simulink library "Displays_Lib"  (Simulink 8.1)
settings: Solver=ode45  StartTime=0.0  StopTime=10.0  RelTol=1e-3
undefined symbols (not defined in the file): ending_column_index, ending_row_index, framebuffer_16x1, framebuffer_2x2, framebuffer_4x4, framebuffer_8x8, HEIGHT, hot, POS_X, POS_Y, starting_column_index, starting_row_index, WIDTH
libraries: dspmtrx3 x119, commutil2 x100, dspsnks4 x4
(part 1 of 2)
settings Model: Creator=uzivatel  LastModifiedBy=uzivatel

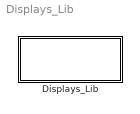
== system Displays_Lib ==
  Displays_Lib : Subsystem

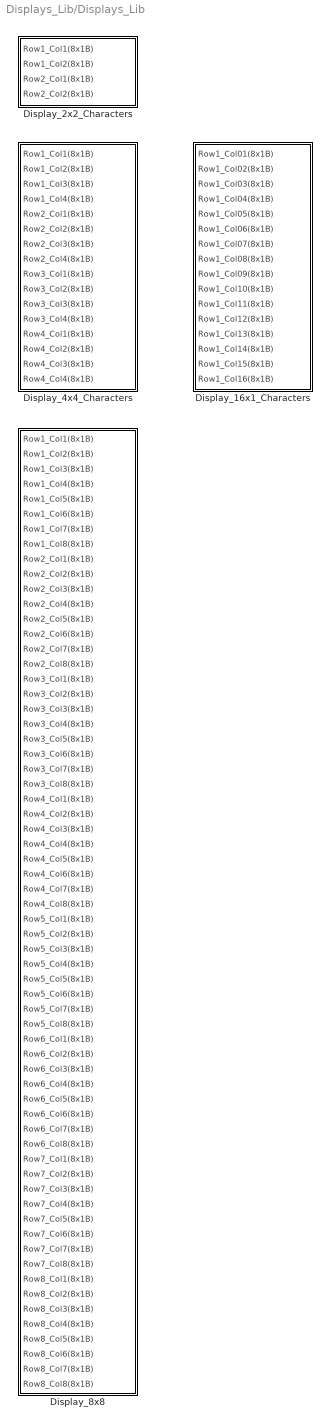
== system Displays_Lib/Displays_Lib ==
  Display_16x1_Characters : Subsystem
  Display_2x2_Characters : Subsystem
  Display_4x4_Characters : Subsystem
  Display_8x8 : Subsystem

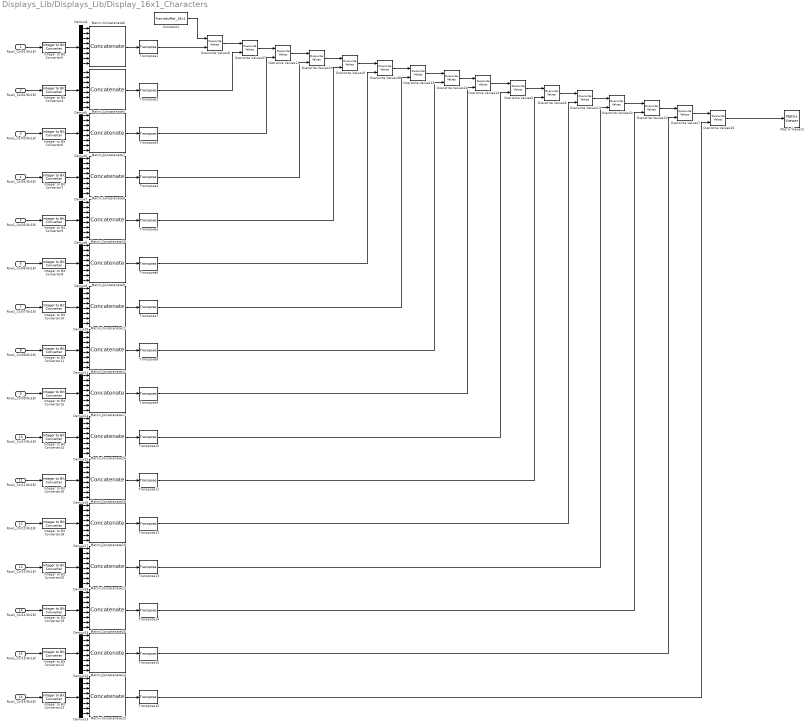
== system Displays_Lib/Displays_Lib/Display_16x1_Characters ==
  Row1_Col01(8x1B) : Inport
  Row1_Col02(8x1B) : Inport  Port=2
  Row1_Col03(8x1B) : Inport  Port=3
  Row1_Col04(8x1B) : Inport  Port=4
  Row1_Col05(8x1B) : Inport  Port=5
  Row1_Col06(8x1B) : Inport  Port=6
  Row1_Col07(8x1B) : Inport  Port=7
  Row1_Col08(8x1B) : Inport  Port=8
  Row1_Col09(8x1B) : Inport  Port=9
  Row1_Col10(8x1B) : Inport  Port=10
  Row1_Col11(8x1B) : Inport  Port=11
  Row1_Col12(8x1B) : Inport  Port=12
  Row1_Col13(8x1B) : Inport  Port=13
  Row1_Col14(8x1B) : Inport  Port=14
  Row1_Col15(8x1B) : Inport  Port=15
  Row1_Col16(8x1B) : Inport  Port=16
  Constant1 : Constant  Value=framebuffer_16x1  OutDataTypeStr=uint8
  Demux{4..19} (16 alike) : Demux  Outputs=8
  Integer to Bit Converter{4..16,18..20} (16 alike) : commutil2/Integer to Bit Converter  nbits=8  signedInputValues=Unsigned  bitOrder=MSB first  outDtype=uint8
  Matrix Concatenate{5..20} (16 alike) : Concatenate  NumInputs=8  Mode=Multidimensional array  ConcatenateDimension=2
  Matrix Viewer2 : dspsnks4/Matrix Viewer  ImageParams=off  CMapStr=[0 0.3 0; 0 1 0]  AxisColorbar=on  AxisParams=off  AxisOrigin=Upper left corner  XLabel=X-axis  YLabel=Y-axis  ZLabel=Z-axis  FigPos=[POS_X POS_Y-140 WIDTH HEIGHT]  AxisZoom=on
      settings: YMin=0  YMax=1
  Overwrite Values10 : dspmtrx3/Overwrite Values  OverWriteDiag=Submatrix  valFrom2ndIP=Second input port  ConstValue=0  RowSpan=Range of rows  RowStartMode=Index  RowStartIndex=starting_row_index(1)  RowEndMode=Index  RowEndIndex=ending_row_index(1)  ColSpan=Range of columns  ColStartMode=Index  ColStartIndex=starting_column_index(14)  ColEndMode=Index  ColEndIndex=ending_column_index(14)  DiagSpan=Range of elements  DiagStartMode=Index  DiagStartIndex=2  DiagEndMode=Index  DiagEndIndex=4
  Overwrite Values11 : dspmtrx3/Overwrite Values  OverWriteDiag=Submatrix  valFrom2ndIP=Second input port  ConstValue=0  RowSpan=Range of rows  RowStartMode=Index  RowStartIndex=starting_row_index(1)  RowEndMode=Index  RowEndIndex=ending_row_index(1)  ColSpan=Range of columns  ColStartMode=Index  ColStartIndex=starting_column_index(3)  ColEndMode=Index  ColEndIndex=ending_column_index(3)  DiagSpan=Range of elements  DiagStartMode=Index  DiagStartIndex=2  DiagEndMode=Index  DiagEndIndex=4
  Overwrite Values12 : dspmtrx3/Overwrite Values  OverWriteDiag=Submatrix  valFrom2ndIP=Second input port  ConstValue=0  RowSpan=Range of rows  RowStartMode=Index  RowStartIndex=starting_row_index(1)  RowEndMode=Index  RowEndIndex=ending_row_index(1)  ColSpan=Range of columns  ColStartMode=Index  ColStartIndex=starting_column_index(7)  ColEndMode=Index  ColEndIndex=ending_column_index(7)  DiagSpan=Range of elements  DiagStartMode=Index  DiagStartIndex=2  DiagEndMode=Index  DiagEndIndex=4
  Overwrite Values13 : dspmtrx3/Overwrite Values  OverWriteDiag=Submatrix  valFrom2ndIP=Second input port  ConstValue=0  RowSpan=Range of rows  RowStartMode=Index  RowStartIndex=starting_row_index(1)  RowEndMode=Index  RowEndIndex=ending_row_index(1)  ColSpan=Range of columns  ColStartMode=Index  ColStartIndex=starting_column_index(12)  ColEndMode=Index  ColEndIndex=ending_column_index(12)  DiagSpan=Range of elements  DiagStartMode=Index  DiagStartIndex=2  DiagEndMode=Index  DiagEndIndex=4
  Overwrite Values14 : dspmtrx3/Overwrite Values  OverWriteDiag=Submatrix  valFrom2ndIP=Second input port  ConstValue=0  RowSpan=Range of rows  RowStartMode=Index  RowStartIndex=starting_row_index(1)  RowEndMode=Index  RowEndIndex=ending_row_index(1)  ColSpan=Range of columns  ColStartMode=Index  ColStartIndex=starting_column_index(9)  ColEndMode=Index  ColEndIndex=ending_column_index(9)  DiagSpan=Range of elements  DiagStartMode=Index  DiagStartIndex=2  DiagEndMode=Index  DiagEndIndex=4
  Overwrite Values16 : dspmtrx3/Overwrite Values  OverWriteDiag=Submatrix  valFrom2ndIP=Second input port  ConstValue=0  RowSpan=Range of rows  RowStartMode=Index  RowStartIndex=starting_row_index(1)  RowEndMode=Index  RowEndIndex=ending_row_index(1)  ColSpan=Range of columns  ColStartMode=Index  ColStartIndex=starting_column_index(16)  ColEndMode=Index  ColEndIndex=ending_column_index(16)  DiagSpan=Range of elements  DiagStartMode=Index  DiagStartIndex=2  DiagEndMode=Index  DiagEndIndex=4
  Overwrite Values20 : dspmtrx3/Overwrite Values  OverWriteDiag=Submatrix  valFrom2ndIP=Second input port  ConstValue=0  RowSpan=Range of rows  RowStartMode=Index  RowStartIndex=starting_row_index(1)  RowEndMode=Index  RowEndIndex=ending_row_index(1)  ColSpan=Range of columns  ColStartMode=Index  ColStartIndex=starting_column_index(13)  ColEndMode=Index  ColEndIndex=ending_column_index(13)  DiagSpan=Range of elements  DiagStartMode=Index  DiagStartIndex=2  DiagEndMode=Index  DiagEndIndex=4
  Overwrite Values23 : dspmtrx3/Overwrite Values  OverWriteDiag=Submatrix  valFrom2ndIP=Second input port  ConstValue=0  RowSpan=Range of rows  RowStartMode=Index  RowStartIndex=starting_row_index(1)  RowEndMode=Index  RowEndIndex=ending_row_index(1)  ColSpan=Range of columns  ColStartMode=Index  ColStartIndex=starting_column_index(4)  ColEndMode=Index  ColEndIndex=ending_column_index(4)  DiagSpan=Range of elements  DiagStartMode=Index  DiagStartIndex=2  DiagEndMode=Index  DiagEndIndex=4
  Overwrite Values24 : dspmtrx3/Overwrite Values  OverWriteDiag=Submatrix  valFrom2ndIP=Second input port  ConstValue=0  RowSpan=Range of rows  RowStartMode=Index  RowStartIndex=starting_row_index(1)  RowEndMode=Index  RowEndIndex=ending_row_index(1)  ColSpan=Range of columns  ColStartMode=Index  ColStartIndex=starting_column_index(8)  ColEndMode=Index  ColEndIndex=ending_column_index(8)  DiagSpan=Range of elements  DiagStartMode=Index  DiagStartIndex=2  DiagEndMode=Index  DiagEndIndex=4
  Overwrite Values37 : dspmtrx3/Overwrite Values  OverWriteDiag=Submatrix  valFrom2ndIP=Second input port  ConstValue=0  RowSpan=Range of rows  RowStartMode=Index  RowStartIndex=starting_row_index(1)  RowEndMode=Index  RowEndIndex=ending_row_index(1)  ColSpan=Range of columns  ColStartMode=Index  ColStartIndex=starting_column_index(2)  ColEndMode=Index  ColEndIndex=ending_column_index(2)  DiagSpan=Range of elements  DiagStartMode=Index  DiagStartIndex=2  DiagEndMode=Index  DiagEndIndex=4
  Overwrite Values38 : dspmtrx3/Overwrite Values  OverWriteDiag=Submatrix  valFrom2ndIP=Second input port  ConstValue=0  RowSpan=Range of rows  RowStartMode=Index  RowStartIndex=starting_row_index(1)  RowEndMode=Index  RowEndIndex=ending_row_index(1)  ColSpan=Range of columns  ColStartMode=Index  ColStartIndex=starting_column_index(6)  ColEndMode=Index  ColEndIndex=ending_column_index(6)  DiagSpan=Range of elements  DiagStartMode=Index  DiagStartIndex=2  DiagEndMode=Index  DiagEndIndex=4
  Overwrite Values5 : dspmtrx3/Overwrite Values  OverWriteDiag=Submatrix  valFrom2ndIP=Second input port  ConstValue=0  RowSpan=Range of rows  RowStartMode=Index  RowStartIndex=starting_row_index(1)  RowEndMode=Index  RowEndIndex=ending_row_index(1)  ColSpan=Range of columns  ColStartMode=Index  ColStartIndex=starting_column_index(10)  ColEndMode=Index  ColEndIndex=ending_column_index(10)  DiagSpan=Range of elements  DiagStartMode=Index  DiagStartIndex=2  DiagEndMode=Index  DiagEndIndex=4
  Overwrite Values6 : dspmtrx3/Overwrite Values  OverWriteDiag=Submatrix  valFrom2ndIP=Second input port  ConstValue=0  RowSpan=Range of rows  RowStartMode=Index  RowStartIndex=starting_row_index(1)  RowEndMode=Index  RowEndIndex=ending_row_index(1)  ColSpan=Range of columns  ColStartMode=Index  ColStartIndex=starting_column_index(11)  ColEndMode=Index  ColEndIndex=ending_column_index(11)  DiagSpan=Range of elements  DiagStartMode=Index  DiagStartIndex=2  DiagEndMode=Index  DiagEndIndex=4
  Overwrite Values7 : dspmtrx3/Overwrite Values  OverWriteDiag=Submatrix  valFrom2ndIP=Second input port  ConstValue=0  RowSpan=Range of rows  RowStartMode=Index  RowStartIndex=starting_row_index(1)  RowEndMode=Index  RowEndIndex=ending_row_index(1)  ColSpan=Range of columns  ColStartMode=Index  ColStartIndex=starting_column_index(15)  ColEndMode=Index  ColEndIndex=ending_column_index(15)  DiagSpan=Range of elements  DiagStartMode=Index  DiagStartIndex=2  DiagEndMode=Index  DiagEndIndex=4
  Overwrite Values8 : dspmtrx3/Overwrite Values  OverWriteDiag=Submatrix  valFrom2ndIP=Second input port  ConstValue=0  RowSpan=Range of rows  RowStartMode=Index  RowStartIndex=starting_row_index(1)  RowEndMode=Index  RowEndIndex=ending_row_index(1)  ColSpan=Range of columns  ColStartMode=Index  ColStartIndex=starting_column_index(1)  ColEndMode=Index  ColEndIndex=ending_column_index(1)  DiagSpan=Range of elements  DiagStartMode=Index  DiagStartIndex=2  DiagEndMode=Index  DiagEndIndex=4
  Overwrite Values9 : dspmtrx3/Overwrite Values  OverWriteDiag=Submatrix  valFrom2ndIP=Second input port  ConstValue=0  RowSpan=Range of rows  RowStartMode=Index  RowStartIndex=starting_row_index(1)  RowEndMode=Index  RowEndIndex=ending_row_index(1)  ColSpan=Range of columns  ColStartMode=Index  ColStartIndex=starting_column_index(5)  ColEndMode=Index  ColEndIndex=ending_column_index(5)  DiagSpan=Range of elements  DiagStartMode=Index  DiagStartIndex=2  DiagEndMode=Index  DiagEndIndex=4
  Transpose{1..16} (16 alike) : dspmtrx3/Transpose  Hermitian=off  overflowFlag=off
  wires:
  Overwrite Values7/1 -> Overwrite Values16/1
  Transpose11/1 -> Overwrite Values6/2
  Transpose13/1 -> Overwrite Values20/2
  Transpose12/1 -> Overwrite Values13/2
  Demux8/8 -> Matrix Concatenate10/8
  Row1_Col05(8x1B)/1 -> Integer to Bit Converter9/1
  Integer to Bit Converter9/1 -> Demux8/1
  Demux9/4 -> Matrix Concatenate9/4
  Integer to Bit Converter11/1 -> Demux11/1
  Demux10/6 -> Matrix Concatenate11/6
  Row1_Col06(8x1B)/1 -> Integer to Bit Converter8/1
  Demux9/7 -> Matrix Concatenate9/7
  Demux11/1 -> Matrix Concatenate12/1
  Demux10/4 -> Matrix Concatenate11/4
  Demux9/2 -> Matrix Concatenate9/2
  Demux11/7 -> Matrix Concatenate12/7
  Demux10/8 -> Matrix Concatenate11/8
  Demux11/4 -> Matrix Concatenate12/4
  Demux9/5 -> Matrix Concatenate9/5
  Demux11/2 -> Matrix Concatenate12/2
  Demux11/5 -> Matrix Concatenate12/5
  Demux11/6 -> Matrix Concatenate12/6
  Row1_Col08(8x1B)/1 -> Integer to Bit Converter11/1
  Demux10/3 -> Matrix Concatenate11/3
  Demux8/2 -> Matrix Concatenate10/2
  Demux8/7 -> Matrix Concatenate10/7
  Overwrite Values24/1 -> Overwrite Values14/1
  Demux10/1 -> Matrix Concatenate11/1
  Demux9/6 -> Matrix Concatenate9/6
  Row1_Col07(8x1B)/1 -> Integer to Bit Converter10/1
  Demux9/8 -> Matrix Concatenate9/8
  Demux10/7 -> Matrix Concatenate11/7
  Demux9/3 -> Matrix Concatenate9/3
  Demux10/2 -> Matrix Concatenate11/2
  Demux11/8 -> Matrix Concatenate12/8
  Demux8/1 -> Matrix Concatenate10/1
  Integer to Bit Converter8/1 -> Demux9/1
  Demux8/5 -> Matrix Concatenate10/5
  Integer to Bit Converter10/1 -> Demux10/1
  Demux11/3 -> Matrix Concatenate12/3
  Demux10/5 -> Matrix Concatenate11/5
  Demux8/6 -> Matrix Concatenate10/6
  Demux8/4 -> Matrix Concatenate10/4
  Demux8/3 -> Matrix Concatenate10/3
  Demux9/1 -> Matrix Concatenate9/1
  Transpose2/1 -> Overwrite Values37/2
  Transpose16/1 -> Overwrite Values16/2
  Transpose14/1 -> Overwrite Values10/2
  Transpose15/1 -> Overwrite Values7/2
  Overwrite Values9/1 -> Overwrite Values38/1
  Overwrite Values6/1 -> Overwrite Values13/1
  Overwrite Values38/1 -> Overwrite Values12/1
  Overwrite Values12/1 -> Overwrite Values24/1
  Overwrite Values14/1 -> Overwrite Values5/1
  Transpose10/1 -> Overwrite Values5/2
  Overwrite Values10/1 -> Overwrite Values7/1
  Integer to Bit Converter18/1 -> Demux17/1
  Transpose5/1 -> Overwrite Values9/2
  Transpose7/1 -> Overwrite Values12/2
  Transpose9/1 -> Overwrite Values14/2
  Transpose4/1 -> Overwrite Values23/2
  Transpose3/1 -> Overwrite Values11/2
  Overwrite Values5/1 -> Overwrite Values6/1
  Overwrite Values20/1 -> Overwrite Values10/1
  Overwrite Values8/1 -> Overwrite Values37/1
  Transpose8/1 -> Overwrite Values24/2
  Demux15/2 -> Matrix Concatenate16/2
  Demux14/3 -> Matrix Concatenate17/3
  Transpose6/1 -> Overwrite Values38/2
  Demux16/1 -> Matrix Concatenate18/1
  Demux15/3 -> Matrix Concatenate16/3
  Overwrite Values11/1 -> Overwrite Values23/1
  Demux15/7 -> Matrix Concatenate16/7
  Demux16/4 -> Matrix Concatenate18/4
  Integer to Bit Converter16/1 -> Demux16/1
  Demux14/1 -> Matrix Concatenate17/1
  Demux15/6 -> Matrix Concatenate16/6
  Demux16/3 -> Matrix Concatenate18/3
  Demux14/4 -> Matrix Concatenate17/4
  Demux16/7 -> Matrix Concatenate18/7
  Demux17/6 -> Matrix Concatenate19/6
  Demux15/5 -> Matrix Concatenate16/5
  Demux14/2 -> Matrix Concatenate17/2
  Demux16/6 -> Matrix Concatenate18/6
  Demux17/7 -> Matrix Concatenate19/7
  Demux16/2 -> Matrix Concatenate18/2
  Demux17/4 -> Matrix Concatenate19/4
  Integer to Bit Converter14/1 -> Demux15/1
  Demux16/5 -> Matrix Concatenate18/5
  Demux15/4 -> Matrix Concatenate16/4
  Demux15/1 -> Matrix Concatenate16/1
  Demux17/5 -> Matrix Concatenate19/5
  Demux19/7 -> Matrix Concatenate20/7
  Integer to Bit Converter19/1 -> Demux19/1
  Demux18/1 -> Matrix Concatenate13/1
  Demux18/2 -> Matrix Concatenate13/2
  Demux18/3 -> Matrix Concatenate13/3
  Demux18/4 -> Matrix Concatenate13/4
  Demux18/5 -> Matrix Concatenate13/5
  Demux18/6 -> Matrix Concatenate13/6
  Demux18/7 -> Matrix Concatenate13/7
  Demux18/8 -> Matrix Concatenate13/8
  Integer to Bit Converter20/1 -> Demux18/1
  Row1_Col13(8x1B)/1 -> Integer to Bit Converter20/1
  Row1_Col15(8x1B)/1 -> Integer to Bit Converter12/1
  Row1_Col14(8x1B)/1 -> Integer to Bit Converter19/1
  Row1_Col16(8x1B)/1 -> Integer to Bit Converter13/1
  Demux17/8 -> Matrix Concatenate19/8
  Demux16/8 -> Matrix Concatenate18/8
  Demux15/8 -> Matrix Concatenate16/8
  Demux17/1 -> Matrix Concatenate19/1
  Demux17/2 -> Matrix Concatenate19/2
  Demux17/3 -> Matrix Concatenate19/3
  Demux19/6 -> Matrix Concatenate20/6
  Demux13/8 -> Matrix Concatenate15/8
  Demux12/8 -> Matrix Concatenate14/8
  Demux19/8 -> Matrix Concatenate20/8
  Demux13/1 -> Matrix Concatenate15/1
  Demux13/2 -> Matrix Concatenate15/2
  Demux13/3 -> Matrix Concatenate15/3
  Demux13/4 -> Matrix Concatenate15/4
  Demux13/5 -> Matrix Concatenate15/5
  Demux13/6 -> Matrix Concatenate15/6
  Demux13/7 -> Matrix Concatenate15/7
  Integer to Bit Converter13/1 -> Demux13/1
  Demux12/1 -> Matrix Concatenate14/1
  Demux12/2 -> Matrix Concatenate14/2
  Demux12/3 -> Matrix Concatenate14/3
  Demux12/4 -> Matrix Concatenate14/4
  Demux12/5 -> Matrix Concatenate14/5
  Demux12/6 -> Matrix Concatenate14/6
  Demux12/7 -> Matrix Concatenate14/7
  Integer to Bit Converter12/1 -> Demux12/1
  Demux19/1 -> Matrix Concatenate20/1
  Demux19/2 -> Matrix Concatenate20/2
  Demux19/3 -> Matrix Concatenate20/3
  Demux19/4 -> Matrix Concatenate20/4
  Demux19/5 -> Matrix Concatenate20/5
  Overwrite Values13/1 -> Overwrite Values20/1
  Demux14/6 -> Matrix Concatenate17/6
  Overwrite Values16/1 -> Matrix Viewer2/1
  Row1_Col09(8x1B)/1 -> Integer to Bit Converter15/1
  Row1_Col11(8x1B)/1 -> Integer to Bit Converter16/1
  Demux14/8 -> Matrix Concatenate17/8
  Constant1/1 -> Overwrite Values8/1
  Row1_Col10(8x1B)/1 -> Integer to Bit Converter14/1
  Demux14/5 -> Matrix Concatenate17/5
  Demux14/7 -> Matrix Concatenate17/7
  Integer to Bit Converter15/1 -> Demux14/1
  Transpose1/1 -> Overwrite Values8/2
  Row1_Col12(8x1B)/1 -> Integer to Bit Converter18/1
  Demux6/2 -> Matrix Concatenate7/2
  Demux6/4 -> Matrix Concatenate7/4
  Demux6/3 -> Matrix Concatenate7/3
  Integer to Bit Converter5/1 -> Demux4/1
  Demux6/1 -> Matrix Concatenate7/1
  Demux6/5 -> Matrix Concatenate7/5
  Demux6/6 -> Matrix Concatenate7/6
  Demux6/7 -> Matrix Concatenate7/7
  Demux4/2 -> Matrix Concatenate6/2
  Row1_Col01(8x1B)/1 -> Integer to Bit Converter5/1
  Integer to Bit Converter7/1 -> Demux7/1
  Demux7/4 -> Matrix Concatenate8/4
  Demux4/4 -> Matrix Concatenate6/4
  Integer to Bit Converter6/1 -> Demux6/1
  Demux4/8 -> Matrix Concatenate6/8
  Demux4/1 -> Matrix Concatenate6/1
  Integer to Bit Converter4/1 -> Demux5/1
  Demux4/7 -> Matrix Concatenate6/7
  Demux4/6 -> Matrix Concatenate6/6
  Demux4/5 -> Matrix Concatenate6/5
  Row1_Col02(8x1B)/1 -> Integer to Bit Converter4/1
  Demux5/4 -> Matrix Concatenate5/4
  Demux5/3 -> Matrix Concatenate5/3
  Demux5/6 -> Matrix Concatenate5/6
  Demux5/8 -> Matrix Concatenate5/8
  Demux5/1 -> Matrix Concatenate5/1
  Demux7/7 -> Matrix Concatenate8/7
  Demux5/2 -> Matrix Concatenate5/2
  Demux7/2 -> Matrix Concatenate8/2
  Demux7/3 -> Matrix Concatenate8/3
  Demux7/8 -> Matrix Concatenate8/8
  Demux6/8 -> Matrix Concatenate7/8
  Demux7/5 -> Matrix Concatenate8/5
  Demux7/6 -> Matrix Concatenate8/6
  Demux7/1 -> Matrix Concatenate8/1
  Demux5/5 -> Matrix Concatenate5/5
  Demux4/3 -> Matrix Concatenate6/3
  Demux5/7 -> Matrix Concatenate5/7
  Row1_Col04(8x1B)/1 -> Integer to Bit Converter7/1
  Row1_Col03(8x1B)/1 -> Integer to Bit Converter6/1
  Overwrite Values23/1 -> Overwrite Values9/1
  Overwrite Values37/1 -> Overwrite Values11/1
  Matrix Concatenate6/1 -> Transpose1/1
  Matrix Concatenate5/1 -> Transpose2/1
  Matrix Concatenate7/1 -> Transpose3/1
  Matrix Concatenate8/1 -> Transpose4/1
  Matrix Concatenate10/1 -> Transpose5/1
  Matrix Concatenate9/1 -> Transpose6/1
  Matrix Concatenate11/1 -> Transpose7/1
  Matrix Concatenate12/1 -> Transpose8/1
  Matrix Concatenate17/1 -> Transpose9/1
  Matrix Concatenate16/1 -> Transpose10/1
  Matrix Concatenate18/1 -> Transpose11/1
  Matrix Concatenate19/1 -> Transpose12/1
  Matrix Concatenate13/1 -> Transpose13/1
  Matrix Concatenate20/1 -> Transpose14/1
  Matrix Concatenate14/1 -> Transpose15/1
  Matrix Concatenate15/1 -> Transpose16/1

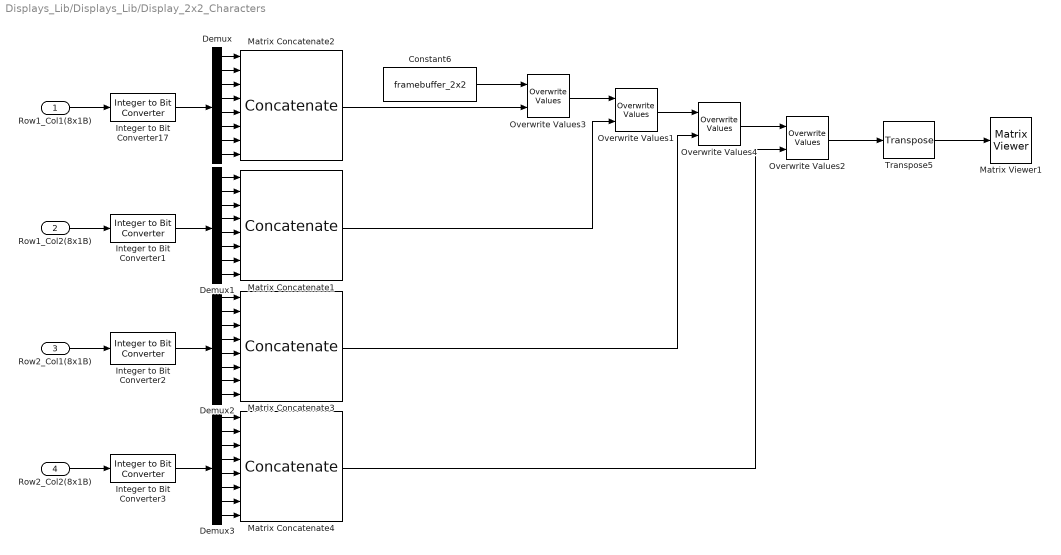
== system Displays_Lib/Displays_Lib/Display_2x2_Characters ==
  Row1_Col1(8x1B) : Inport
  Row1_Col2(8x1B) : Inport  Port=2
  Row2_Col1(8x1B) : Inport  Port=3
  Row2_Col2(8x1B) : Inport  Port=4
  Constant6 : Constant  Value=framebuffer_2x2  OutDataTypeStr=uint8
  Demux{,1..3} (4 alike) : Demux  Outputs=8
  Integer to Bit Converter{1..3,17} (4 alike) : commutil2/Integer to Bit Converter  nbits=8  signedInputValues=Unsigned  bitOrder=MSB first  outDtype=uint8
  Matrix Concatenate{1..4} (4 alike) : Concatenate  NumInputs=8  Mode=Multidimensional array  ConcatenateDimension=2
  Matrix Viewer1 : dspsnks4/Matrix Viewer  ImageParams=off  CMapStr=hot(256)  AxisColorbar=on  AxisParams=off  AxisOrigin=Upper left corner  XLabel=X-axis  YLabel=Y-axis  ZLabel=Z-axis  FigPos=[POS_X POS_Y-140 WIDTH HEIGHT]  AxisZoom=on
      settings: YMin=0  YMax=1.0
  Overwrite Values1 : dspmtrx3/Overwrite Values  OverWriteDiag=Submatrix  valFrom2ndIP=Second input port  ConstValue=0  RowSpan=Range of rows  RowStartMode=Index  RowStartIndex=starting_row_index(1)  RowEndMode=Index  RowEndIndex=ending_row_index(1)  ColSpan=Range of columns  ColStartMode=Index  ColStartIndex=starting_column_index(2)  ColEndMode=Index  ColEndIndex=ending_column_index(2)  DiagSpan=Range of elements  DiagStartMode=Index  DiagStartIndex=2  DiagEndMode=Index  DiagEndIndex=4
  Overwrite Values2 : dspmtrx3/Overwrite Values  OverWriteDiag=Submatrix  valFrom2ndIP=Second input port  ConstValue=0  RowSpan=Range of rows  RowStartMode=Index  RowStartIndex=starting_row_index(2)  RowEndMode=Index  RowEndIndex=ending_row_index(2)  ColSpan=Range of columns  ColStartMode=Index  ColStartIndex=starting_column_index(2)  ColEndMode=Index  ColEndIndex=ending_column_index(2)  DiagSpan=Range of elements  DiagStartMode=Index  DiagStartIndex=2  DiagEndMode=Index  DiagEndIndex=4
  Overwrite Values3 : dspmtrx3/Overwrite Values  OverWriteDiag=Submatrix  valFrom2ndIP=Second input port  ConstValue=0  RowSpan=Range of rows  RowStartMode=Index  RowStartIndex=starting_row_index(1)  RowEndMode=Index  RowEndIndex=ending_row_index(1)  ColSpan=Range of columns  ColStartMode=Index  ColStartIndex=starting_column_index(1)  ColEndMode=Index  ColEndIndex=ending_column_index(1)  DiagSpan=Range of elements  DiagStartMode=Index  DiagStartIndex=2  DiagEndMode=Index  DiagEndIndex=4
  Overwrite Values4 : dspmtrx3/Overwrite Values  OverWriteDiag=Submatrix  valFrom2ndIP=Second input port  ConstValue=0  RowSpan=Range of rows  RowStartMode=Index  RowStartIndex=starting_row_index(2)  RowEndMode=Index  RowEndIndex=ending_row_index(2)  ColSpan=Range of columns  ColStartMode=Index  ColStartIndex=starting_column_index(1)  ColEndMode=Index  ColEndIndex=ending_column_index(1)  DiagSpan=Range of elements  DiagStartMode=Index  DiagStartIndex=2  DiagEndMode=Index  DiagEndIndex=4
  Transpose5 : dspmtrx3/Transpose  Hermitian=off  overflowFlag=off
  wires:
  Transpose5/1 -> Matrix Viewer1/1
  Matrix Concatenate4/1 -> Overwrite Values2/2
  Demux3/8 -> Matrix Concatenate4/8
  Demux2/8 -> Matrix Concatenate3/8
  Matrix Concatenate3/1 -> Overwrite Values4/2
  Matrix Concatenate1/1 -> Overwrite Values1/2
  Demux1/8 -> Matrix Concatenate1/8
  Demux3/1 -> Matrix Concatenate4/1
  Demux3/2 -> Matrix Concatenate4/2
  Demux3/3 -> Matrix Concatenate4/3
  Demux3/4 -> Matrix Concatenate4/4
  Demux3/5 -> Matrix Concatenate4/5
  Demux3/6 -> Matrix Concatenate4/6
  Demux3/7 -> Matrix Concatenate4/7
  Integer to Bit Converter3/1 -> Demux3/1
  Demux2/1 -> Matrix Concatenate3/1
  Demux2/2 -> Matrix Concatenate3/2
  Demux2/3 -> Matrix Concatenate3/3
  Demux2/4 -> Matrix Concatenate3/4
  Demux2/5 -> Matrix Concatenate3/5
  Demux2/6 -> Matrix Concatenate3/6
  Demux2/7 -> Matrix Concatenate3/7
  Integer to Bit Converter2/1 -> Demux2/1
  Demux1/1 -> Matrix Concatenate1/1
  Demux1/2 -> Matrix Concatenate1/2
  Demux1/3 -> Matrix Concatenate1/3
  Demux1/4 -> Matrix Concatenate1/4
  Demux1/5 -> Matrix Concatenate1/5
  Demux1/6 -> Matrix Concatenate1/6
  Demux1/7 -> Matrix Concatenate1/7
  Integer to Bit Converter1/1 -> Demux1/1
  Matrix Concatenate2/1 -> Overwrite Values3/2
  Demux/1 -> Matrix Concatenate2/1
  Demux/2 -> Matrix Concatenate2/2
  Demux/3 -> Matrix Concatenate2/3
  Demux/4 -> Matrix Concatenate2/4
  Demux/5 -> Matrix Concatenate2/5
  Demux/6 -> Matrix Concatenate2/6
  Demux/7 -> Matrix Concatenate2/7
  Demux/8 -> Matrix Concatenate2/8
  Integer to Bit Converter17/1 -> Demux/1
  Row1_Col1(8x1B)/1 -> Integer to Bit Converter17/1
  Overwrite Values1/1 -> Overwrite Values4/1
  Row2_Col1(8x1B)/1 -> Integer to Bit Converter2/1
  Overwrite Values4/1 -> Overwrite Values2/1
  Constant6/1 -> Overwrite Values3/1
  Overwrite Values3/1 -> Overwrite Values1/1
  Row1_Col2(8x1B)/1 -> Integer to Bit Converter1/1
  Row2_Col2(8x1B)/1 -> Integer to Bit Converter3/1
  Overwrite Values2/1 -> Transpose5/1

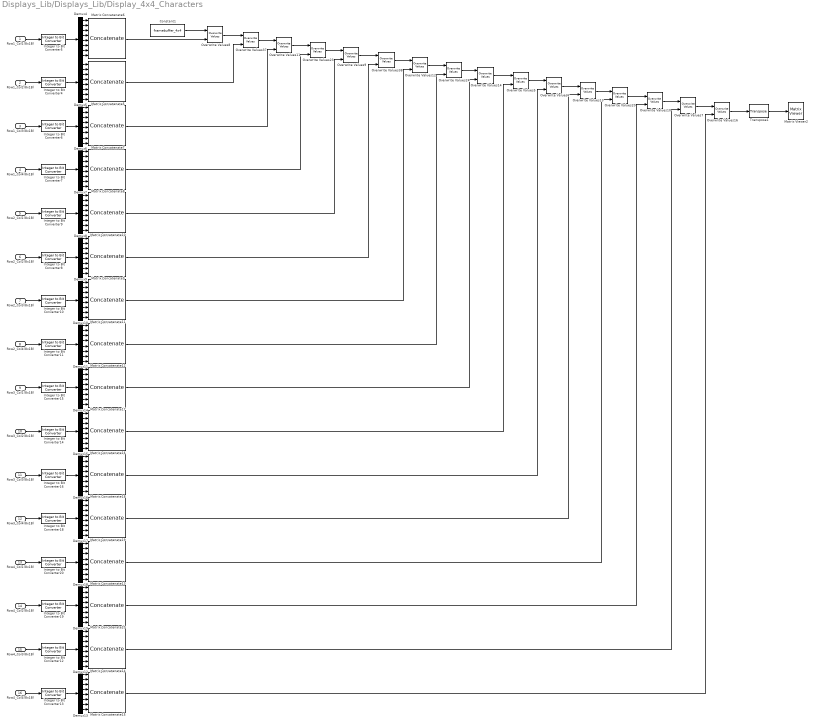
== system Displays_Lib/Displays_Lib/Display_4x4_Characters ==
  Row1_Col1(8x1B) : Inport
  Row1_Col2(8x1B) : Inport  Port=2
  Row1_Col3(8x1B) : Inport  Port=3
  Row1_Col4(8x1B) : Inport  Port=4
  Row2_Col1(8x1B) : Inport  Port=5
  Row2_Col2(8x1B) : Inport  Port=6
  Row2_Col3(8x1B) : Inport  Port=7
  Row2_Col4(8x1B) : Inport  Port=8
  Row3_Col1(8x1B) : Inport  Port=9
  Row3_Col2(8x1B) : Inport  Port=10
  Row3_Col3(8x1B) : Inport  Port=11
  Row3_Col4(8x1B) : Inport  Port=12
  Row4_Col1(8x1B) : Inport  Port=13
  Row4_Col2(8x1B) : Inport  Port=14
  Row4_Col3(8x1B) : Inport  Port=15
  Row4_Col4(8x1B) : Inport  Port=16
  Constant1 : Constant  Value=framebuffer_4x4  OutDataTypeStr=uint8
  Demux{4..19} (16 alike) : Demux  Outputs=8
  Integer to Bit Converter{4..16,18..20} (16 alike) : commutil2/Integer to Bit Converter  nbits=8  signedInputValues=Unsigned  bitOrder=MSB first  outDtype=uint8
  Matrix Concatenate{5..20} (16 alike) : Concatenate  NumInputs=8  Mode=Multidimensional array  ConcatenateDimension=2
  Matrix Viewer2 : dspsnks4/Matrix Viewer  ImageParams=off  CMapStr=hot(256)  AxisColorbar=on  AxisParams=off  AxisOrigin=Upper left corner  XLabel=X-axis  YLabel=Y-axis  ZLabel=Z-axis  FigPos=[POS_X POS_Y-140 WIDTH HEIGHT]  AxisZoom=on
      settings: YMin=0  YMax=1.0
  Overwrite Values10 : dspmtrx3/Overwrite Values  OverWriteDiag=Submatrix  valFrom2ndIP=Second input port  ConstValue=0  RowSpan=Range of rows  RowStartMode=Index  RowStartIndex=starting_row_index(4)  RowEndMode=Index  RowEndIndex=ending_row_index(4)  ColSpan=Range of columns  ColStartMode=Index  ColStartIndex=starting_column_index(2)  ColEndMode=Index  ColEndIndex=ending_column_index(2)  DiagSpan=Range of elements  DiagStartMode=Index  DiagStartIndex=2  DiagEndMode=Index  DiagEndIndex=4
  Overwrite Values11 : dspmtrx3/Overwrite Values  OverWriteDiag=Submatrix  valFrom2ndIP=Second input port  ConstValue=0  RowSpan=Range of rows  RowStartMode=Index  RowStartIndex=starting_row_index(1)  RowEndMode=Index  RowEndIndex=ending_row_index(1)  ColSpan=Range of columns  ColStartMode=Index  ColStartIndex=starting_column_index(3)  ColEndMode=Index  ColEndIndex=ending_column_index(3)  DiagSpan=Range of elements  DiagStartMode=Index  DiagStartIndex=2  DiagEndMode=Index  DiagEndIndex=4
  Overwrite Values12 : dspmtrx3/Overwrite Values  OverWriteDiag=Submatrix  valFrom2ndIP=Second input port  ConstValue=0  RowSpan=Range of rows  RowStartMode=Index  RowStartIndex=starting_row_index(2)  RowEndMode=Index  RowEndIndex=ending_row_index(2)  ColSpan=Range of columns  ColStartMode=Index  ColStartIndex=starting_column_index(3)  ColEndMode=Index  ColEndIndex=ending_column_index(3)  DiagSpan=Range of elements  DiagStartMode=Index  DiagStartIndex=2  DiagEndMode=Index  DiagEndIndex=4
  Overwrite Values13 : dspmtrx3/Overwrite Values  OverWriteDiag=Submatrix  valFrom2ndIP=Second input port  ConstValue=0  RowSpan=Range of rows  RowStartMode=Index  RowStartIndex=starting_row_index(3)  RowEndMode=Index  RowEndIndex=ending_row_index(3)  ColSpan=Range of columns  ColStartMode=Index  ColStartIndex=starting_column_index(4)  ColEndMode=Index  ColEndIndex=ending_column_index(4)  DiagSpan=Range of elements  DiagStartMode=Index  DiagStartIndex=2  DiagEndMode=Index  DiagEndIndex=4
  Overwrite Values14 : dspmtrx3/Overwrite Values  OverWriteDiag=Submatrix  valFrom2ndIP=Second input port  ConstValue=0  RowSpan=Range of rows  RowStartMode=Index  RowStartIndex=starting_row_index(3)  RowEndMode=Index  RowEndIndex=ending_row_index(3)  ColSpan=Range of columns  ColStartMode=Index  ColStartIndex=starting_column_index(1)  ColEndMode=Index  ColEndIndex=ending_column_index(1)  DiagSpan=Range of elements  DiagStartMode=Index  DiagStartIndex=2  DiagEndMode=Index  DiagEndIndex=4
  Overwrite Values16 : dspmtrx3/Overwrite Values  OverWriteDiag=Submatrix  valFrom2ndIP=Second input port  ConstValue=0  RowSpan=Range of rows  RowStartMode=Index  RowStartIndex=starting_row_index(4)  RowEndMode=Index  RowEndIndex=ending_row_index(4)  ColSpan=Range of columns  ColStartMode=Index  ColStartIndex=starting_column_index(4)  ColEndMode=Index  ColEndIndex=ending_column_index(4)  DiagSpan=Range of elements  DiagStartMode=Index  DiagStartIndex=2  DiagEndMode=Index  DiagEndIndex=4
  Overwrite Values20 : dspmtrx3/Overwrite Values  OverWriteDiag=Submatrix  valFrom2ndIP=Second input port  ConstValue=0  RowSpan=Range of rows  RowStartMode=Index  RowStartIndex=starting_row_index(4)  RowEndMode=Index  RowEndIndex=ending_row_index(4)  ColSpan=Range of columns  ColStartMode=Index  ColStartIndex=starting_column_index(1)  ColEndMode=Index  ColEndIndex=ending_column_index(1)  DiagSpan=Range of elements  DiagStartMode=Index  DiagStartIndex=2  DiagEndMode=Index  DiagEndIndex=4
  Overwrite Values23 : dspmtrx3/Overwrite Values  OverWriteDiag=Submatrix  valFrom2ndIP=Second input port  ConstValue=0  RowSpan=Range of rows  RowStartMode=Index  RowStartIndex=starting_row_index(1)  RowEndMode=Index  RowEndIndex=ending_row_index(1)  ColSpan=Range of columns  ColStartMode=Index  ColStartIndex=starting_column_index(4)  ColEndMode=Index  ColEndIndex=ending_column_index(4)  DiagSpan=Range of elements  DiagStartMode=Index  DiagStartIndex=2  DiagEndMode=Index  DiagEndIndex=4
  Overwrite Values24 : dspmtrx3/Overwrite Values  OverWriteDiag=Submatrix  valFrom2ndIP=Second input port  ConstValue=0  RowSpan=Range of rows  RowStartMode=Index  RowStartIndex=starting_row_index(2)  RowEndMode=Index  RowEndIndex=ending_row_index(2)  ColSpan=Range of columns  ColStartMode=Index  ColStartIndex=starting_column_index(4)  ColEndMode=Index  ColEndIndex=ending_column_index(4)  DiagSpan=Range of elements  DiagStartMode=Index  DiagStartIndex=2  DiagEndMode=Index  DiagEndIndex=4
  Overwrite Values37 : dspmtrx3/Overwrite Values  OverWriteDiag=Submatrix  valFrom2ndIP=Second input port  ConstValue=0  RowSpan=Range of rows  RowStartMode=Index  RowStartIndex=starting_row_index(1)  RowEndMode=Index  RowEndIndex=ending_row_index(1)  ColSpan=Range of columns  ColStartMode=Index  ColStartIndex=starting_column_index(2)  ColEndMode=Index  ColEndIndex=ending_column_index(2)  DiagSpan=Range of elements  DiagStartMode=Index  DiagStartIndex=2  DiagEndMode=Index  DiagEndIndex=4
  Overwrite Values38 : dspmtrx3/Overwrite Values  OverWriteDiag=Submatrix  valFrom2ndIP=Second input port  ConstValue=0  RowSpan=Range of rows  RowStartMode=Index  RowStartIndex=starting_row_index(2)  RowEndMode=Index  RowEndIndex=ending_row_index(2)  ColSpan=Range of columns  ColStartMode=Index  ColStartIndex=starting_column_index(2)  ColEndMode=Index  ColEndIndex=ending_column_index(2)  DiagSpan=Range of elements  DiagStartMode=Index  DiagStartIndex=2  DiagEndMode=Index  DiagEndIndex=4
  Overwrite Values5 : dspmtrx3/Overwrite Values  OverWriteDiag=Submatrix  valFrom2ndIP=Second input port  ConstValue=0  RowSpan=Range of rows  RowStartMode=Index  RowStartIndex=starting_row_index(3)  RowEndMode=Index  RowEndIndex=ending_row_index(3)  ColSpan=Range of columns  ColStartMode=Index  ColStartIndex=starting_column_index(2)  ColEndMode=Index  ColEndIndex=ending_column_index(2)  DiagSpan=Range of elements  DiagStartMode=Index  DiagStartIndex=2  DiagEndMode=Index  DiagEndIndex=4
  Overwrite Values6 : dspmtrx3/Overwrite Values  OverWriteDiag=Submatrix  valFrom2ndIP=Second input port  ConstValue=0  RowSpan=Range of rows  RowStartMode=Index  RowStartIndex=starting_row_index(3)  RowEndMode=Index  RowEndIndex=ending_row_index(3)  ColSpan=Range of columns  ColStartMode=Index  ColStartIndex=starting_column_index(3)  ColEndMode=Index  ColEndIndex=ending_column_index(3)  DiagSpan=Range of elements  DiagStartMode=Index  DiagStartIndex=2  DiagEndMode=Index  DiagEndIndex=4
  Overwrite Values7 : dspmtrx3/Overwrite Values  OverWriteDiag=Submatrix  valFrom2ndIP=Second input port  ConstValue=0  RowSpan=Range of rows  RowStartMode=Index  RowStartIndex=starting_row_index(4)  RowEndMode=Index  RowEndIndex=ending_row_index(4)  ColSpan=Range of columns  ColStartMode=Index  ColStartIndex=starting_column_index(3)  ColEndMode=Index  ColEndIndex=ending_column_index(3)  DiagSpan=Range of elements  DiagStartMode=Index  DiagStartIndex=2  DiagEndMode=Index  DiagEndIndex=4
  Overwrite Values8 : dspmtrx3/Overwrite Values  OverWriteDiag=Submatrix  valFrom2ndIP=Second input port  ConstValue=0  RowSpan=Range of rows  RowStartMode=Index  RowStartIndex=starting_row_index(1)  RowEndMode=Index  RowEndIndex=ending_row_index(1)  ColSpan=Range of columns  ColStartMode=Index  ColStartIndex=starting_column_index(1)  ColEndMode=Index  ColEndIndex=ending_column_index(1)  DiagSpan=Range of elements  DiagStartMode=Index  DiagStartIndex=2  DiagEndMode=Index  DiagEndIndex=4
  Overwrite Values9 : dspmtrx3/Overwrite Values  OverWriteDiag=Submatrix  valFrom2ndIP=Second input port  ConstValue=0  RowSpan=Range of rows  RowStartMode=Index  RowStartIndex=starting_row_index(2)  RowEndMode=Index  RowEndIndex=ending_row_index(2)  ColSpan=Range of columns  ColStartMode=Index  ColStartIndex=starting_column_index(1)  ColEndMode=Index  ColEndIndex=ending_column_index(1)  DiagSpan=Range of elements  DiagStartMode=Index  DiagStartIndex=2  DiagEndMode=Index  DiagEndIndex=4
  Transpose1 : dspmtrx3/Transpose  Hermitian=off  overflowFlag=off
  wires:
  Overwrite Values7/1 -> Overwrite Values16/1
  Matrix Concatenate18/1 -> Overwrite Values6/2
  Matrix Concatenate13/1 -> Overwrite Values20/2
  Matrix Concatenate19/1 -> Overwrite Values13/2
  Demux8/8 -> Matrix Concatenate10/8
  Row2_Col1(8x1B)/1 -> Integer to Bit Converter9/1
  Integer to Bit Converter9/1 -> Demux8/1
  Demux9/4 -> Matrix Concatenate9/4
  Integer to Bit Converter11/1 -> Demux11/1
  Demux10/6 -> Matrix Concatenate11/6
  Row2_Col2(8x1B)/1 -> Integer to Bit Converter8/1
  Demux9/7 -> Matrix Concatenate9/7
  Demux11/1 -> Matrix Concatenate12/1
  Demux10/4 -> Matrix Concatenate11/4
  Demux9/2 -> Matrix Concatenate9/2
  Demux11/7 -> Matrix Concatenate12/7
  Demux10/8 -> Matrix Concatenate11/8
  Demux11/4 -> Matrix Concatenate12/4
  Demux9/5 -> Matrix Concatenate9/5
  Demux11/2 -> Matrix Concatenate12/2
  Demux11/5 -> Matrix Concatenate12/5
  Demux11/6 -> Matrix Concatenate12/6
  Row2_Col4(8x1B)/1 -> Integer to Bit Converter11/1
  Demux10/3 -> Matrix Concatenate11/3
  Demux8/2 -> Matrix Concatenate10/2
  Demux8/7 -> Matrix Concatenate10/7
  Overwrite Values24/1 -> Overwrite Values14/1
  Demux10/1 -> Matrix Concatenate11/1
  Demux9/6 -> Matrix Concatenate9/6
  Row2_Col3(8x1B)/1 -> Integer to Bit Converter10/1
  Demux9/8 -> Matrix Concatenate9/8
  Demux10/7 -> Matrix Concatenate11/7
  Demux9/3 -> Matrix Concatenate9/3
  Demux10/2 -> Matrix Concatenate11/2
  Demux11/8 -> Matrix Concatenate12/8
  Demux8/1 -> Matrix Concatenate10/1
  Integer to Bit Converter8/1 -> Demux9/1
  Demux8/5 -> Matrix Concatenate10/5
  Integer to Bit Converter10/1 -> Demux10/1
  Demux11/3 -> Matrix Concatenate12/3
  Demux10/5 -> Matrix Concatenate11/5
  Demux8/6 -> Matrix Concatenate10/6
  Demux8/4 -> Matrix Concatenate10/4
  Demux8/3 -> Matrix Concatenate10/3
  Demux9/1 -> Matrix Concatenate9/1
  Matrix Concatenate5/1 -> Overwrite Values37/2
  Matrix Concatenate15/1 -> Overwrite Values16/2
  Matrix Concatenate20/1 -> Overwrite Values10/2
  Matrix Concatenate14/1 -> Overwrite Values7/2
  Overwrite Values9/1 -> Overwrite Values38/1
  Overwrite Values6/1 -> Overwrite Values13/1
  Overwrite Values38/1 -> Overwrite Values12/1
  Overwrite Values12/1 -> Overwrite Values24/1
  Overwrite Values14/1 -> Overwrite Values5/1
  Matrix Concatenate16/1 -> Overwrite Values5/2
  Overwrite Values10/1 -> Overwrite Values7/1
  Integer to Bit Converter18/1 -> Demux17/1
  Matrix Concatenate10/1 -> Overwrite Values9/2
  Matrix Concatenate11/1 -> Overwrite Values12/2
  Matrix Concatenate17/1 -> Overwrite Values14/2
  Matrix Concatenate8/1 -> Overwrite Values23/2
  Matrix Concatenate7/1 -> Overwrite Values11/2
  Overwrite Values5/1 -> Overwrite Values6/1
  Overwrite Values20/1 -> Overwrite Values10/1
  Overwrite Values8/1 -> Overwrite Values37/1
  Matrix Concatenate12/1 -> Overwrite Values24/2
  Demux15/2 -> Matrix Concatenate16/2
  Demux14/3 -> Matrix Concatenate17/3
  Matrix Concatenate9/1 -> Overwrite Values38/2
  Demux16/1 -> Matrix Concatenate18/1
  Demux15/3 -> Matrix Concatenate16/3
  Overwrite Values11/1 -> Overwrite Values23/1
  Demux15/7 -> Matrix Concatenate16/7
  Demux16/4 -> Matrix Concatenate18/4
  Integer to Bit Converter16/1 -> Demux16/1
  Demux14/1 -> Matrix Concatenate17/1
  Demux15/6 -> Matrix Concatenate16/6
  Demux16/3 -> Matrix Concatenate18/3
  Demux14/4 -> Matrix Concatenate17/4
  Demux16/7 -> Matrix Concatenate18/7
  Demux17/6 -> Matrix Concatenate19/6
  Demux15/5 -> Matrix Concatenate16/5
  Demux14/2 -> Matrix Concatenate17/2
  Demux16/6 -> Matrix Concatenate18/6
  Demux17/7 -> Matrix Concatenate19/7
  Demux16/2 -> Matrix Concatenate18/2
  Demux17/4 -> Matrix Concatenate19/4
  Integer to Bit Converter14/1 -> Demux15/1
  Demux16/5 -> Matrix Concatenate18/5
  Demux15/4 -> Matrix Concatenate16/4
  Demux15/1 -> Matrix Concatenate16/1
  Demux17/5 -> Matrix Concatenate19/5
  Demux19/7 -> Matrix Concatenate20/7
  Integer to Bit Converter19/1 -> Demux19/1
  Demux18/1 -> Matrix Concatenate13/1
  Demux18/2 -> Matrix Concatenate13/2
  Demux18/3 -> Matrix Concatenate13/3
  Demux18/4 -> Matrix Concatenate13/4
  Demux18/5 -> Matrix Concatenate13/5
  Demux18/6 -> Matrix Concatenate13/6
  Demux18/7 -> Matrix Concatenate13/7
  Demux18/8 -> Matrix Concatenate13/8
  Integer to Bit Converter20/1 -> Demux18/1
  Row4_Col1(8x1B)/1 -> Integer to Bit Converter20/1
  Row4_Col3(8x1B)/1 -> Integer to Bit Converter12/1
  Row4_Col2(8x1B)/1 -> Integer to Bit Converter19/1
  Row4_Col4(8x1B)/1 -> Integer to Bit Converter13/1
  Demux17/8 -> Matrix Concatenate19/8
  Demux16/8 -> Matrix Concatenate18/8
  Demux15/8 -> Matrix Concatenate16/8
  Demux17/1 -> Matrix Concatenate19/1
  Demux17/2 -> Matrix Concatenate19/2
  Demux17/3 -> Matrix Concatenate19/3
  Demux19/6 -> Matrix Concatenate20/6
  Demux13/8 -> Matrix Concatenate15/8
  Demux12/8 -> Matrix Concatenate14/8
  Demux19/8 -> Matrix Concatenate20/8
  Demux13/1 -> Matrix Concatenate15/1
  Demux13/2 -> Matrix Concatenate15/2
  Demux13/3 -> Matrix Concatenate15/3
  Demux13/4 -> Matrix Concatenate15/4
  Demux13/5 -> Matrix Concatenate15/5
  Demux13/6 -> Matrix Concatenate15/6
  Demux13/7 -> Matrix Concatenate15/7
  Integer to Bit Converter13/1 -> Demux13/1
  Demux12/1 -> Matrix Concatenate14/1
  Demux12/2 -> Matrix Concatenate14/2
  Demux12/3 -> Matrix Concatenate14/3
  Demux12/4 -> Matrix Concatenate14/4
  Demux12/5 -> Matrix Concatenate14/5
  Demux12/6 -> Matrix Concatenate14/6
  Demux12/7 -> Matrix Concatenate14/7
  Integer to Bit Converter12/1 -> Demux12/1
  Demux19/1 -> Matrix Concatenate20/1
  Demux19/2 -> Matrix Concatenate20/2
  Demux19/3 -> Matrix Concatenate20/3
  Demux19/4 -> Matrix Concatenate20/4
  Demux19/5 -> Matrix Concatenate20/5
  Overwrite Values13/1 -> Overwrite Values20/1
  Demux14/6 -> Matrix Concatenate17/6
  Overwrite Values16/1 -> Transpose1/1
  Transpose1/1 -> Matrix Viewer2/1
  Row3_Col1(8x1B)/1 -> Integer to Bit Converter15/1
  Row3_Col3(8x1B)/1 -> Integer to Bit Converter16/1
  Demux14/8 -> Matrix Concatenate17/8
  Constant1/1 -> Overwrite Values8/1
  Row3_Col2(8x1B)/1 -> Integer to Bit Converter14/1
  Demux14/5 -> Matrix Concatenate17/5
  Demux14/7 -> Matrix Concatenate17/7
  Integer to Bit Converter15/1 -> Demux14/1
  Matrix Concatenate6/1 -> Overwrite Values8/2
  Row3_Col4(8x1B)/1 -> Integer to Bit Converter18/1
  Demux6/2 -> Matrix Concatenate7/2
  Demux6/4 -> Matrix Concatenate7/4
  Demux6/3 -> Matrix Concatenate7/3
  Integer to Bit Converter5/1 -> Demux4/1
  Demux6/1 -> Matrix Concatenate7/1
  Demux6/5 -> Matrix Concatenate7/5
  Demux6/6 -> Matrix Concatenate7/6
  Demux6/7 -> Matrix Concatenate7/7
  Demux4/2 -> Matrix Concatenate6/2
  Row1_Col1(8x1B)/1 -> Integer to Bit Converter5/1
  Integer to Bit Converter7/1 -> Demux7/1
  Demux7/4 -> Matrix Concatenate8/4
  Demux4/4 -> Matrix Concatenate6/4
  Integer to Bit Converter6/1 -> Demux6/1
  Demux4/8 -> Matrix Concatenate6/8
  Demux4/1 -> Matrix Concatenate6/1
  Integer to Bit Converter4/1 -> Demux5/1
  Demux4/7 -> Matrix Concatenate6/7
  Demux4/6 -> Matrix Concatenate6/6
  Demux4/5 -> Matrix Concatenate6/5
  Row1_Col2(8x1B)/1 -> Integer to Bit Converter4/1
  Demux5/4 -> Matrix Concatenate5/4
  Demux5/3 -> Matrix Concatenate5/3
  Demux5/6 -> Matrix Concatenate5/6
  Demux5/8 -> Matrix Concatenate5/8
  Demux5/1 -> Matrix Concatenate5/1
  Demux7/7 -> Matrix Concatenate8/7
  Demux5/2 -> Matrix Concatenate5/2
  Demux7/2 -> Matrix Concatenate8/2
  Demux7/3 -> Matrix Concatenate8/3
  Demux7/8 -> Matrix Concatenate8/8
  Demux6/8 -> Matrix Concatenate7/8
  Demux7/5 -> Matrix Concatenate8/5
  Demux7/6 -> Matrix Concatenate8/6
  Demux7/1 -> Matrix Concatenate8/1
  Demux5/5 -> Matrix Concatenate5/5
  Demux4/3 -> Matrix Concatenate6/3
  Demux5/7 -> Matrix Concatenate5/7
  Row1_Col4(8x1B)/1 -> Integer to Bit Converter7/1
  Row1_Col3(8x1B)/1 -> Integer to Bit Converter6/1
  Overwrite Values23/1 -> Overwrite Values9/1
  Overwrite Values37/1 -> Overwrite Values11/1
